simulink model "Scientific_Calculator"  (R2016a)
settings: Solver=FixedStepDiscrete  StartTime=0.0  StopTime=10.0  RelTol=1e-3
settings Model: Creator=NoteBook  LastModifiedBy=NoteBook
settings OptimizationCC: DefaultParameterBehavior=Inlined  EnableMemcpy=off  OptimizeModelRefInitCode=on  LifeSpan=1
settings DebuggingCC: UnderspecifiedInitializationDetection=Classic  MergeDetectMultiDrivingBlocksExec=none
settings ModelReferenceCC: PropagateSignalLabelsOutOfModel=off
settings RTWCC: SystemTargetFile=ert.tlc  GenCodeOnly=on  TemplateMakefile=ert_default_tmf  GenerateReport=on  IncludeHyperlinkInReport=on  LaunchReport=on  GenerateTraceInfo=on  GenerateTraceReport=on  GenerateTraceReportSl=on  GenerateTraceReportSf=on  GenerateTraceReportEml=on
settings CodeAppCC: ForceParamTrailComments=on  IgnoreCustomStorageClasses=off  OperatorAnnotations=on  SimulinkDataObjDesc=on  SFDataObjDesc=on  MATLABFcnDesc=on  InsertBlockDesc=on  MATLABSourceComments=on
settings ERTTargetCC: GenerateSampleERTMain=on  InlinedParameterPlacement=NonHierarchical  ERTCustomFileTemplate=example_file_process.tlc

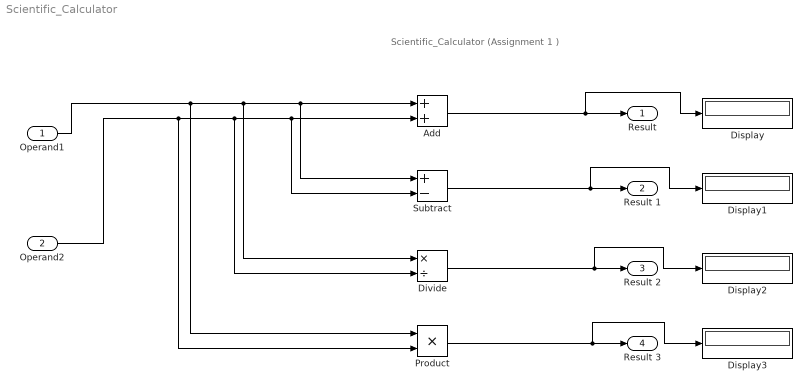
== system Scientific_Calculator ==
  note: Scientific_Calculator (Assignment 1 )
  "Operand1 " : Inport  OutDataTypeStr=uint8
  "Operand2 " : Inport  Port=2  OutDataTypeStr=uint8
  Add : Sum
  Display{,1..3} (4 alike) : Display
  Divide : Product  Inputs=*/
  Product : Product
  Subtract : Sum  Inputs=+-
  "Result " : Outport
  Result 1 : Outport  Port=2
  Result 2 : Outport  Port=3
  Result 3 : Outport  Port=4
  wires:
  "Operand1 "/1 -> Divide/1, Subtract/1, Add/1, Product/1
  "Operand2 "/1 -> Product/2, Divide/2, Subtract/2, Add/2
  Add/1 -> Display/1, "Result "/1
  Subtract/1 -> Display1/1, Result 1/1
  Divide/1 -> Display2/1, Result 2/1
  Product/1 -> Display3/1, Result 3/1
